simulink library "HANcoder_STM32_Target2009b"  (Simulink 7.5)
settings: Solver=ode45  StartTime=0.0  StopTime=10.0  RelTol=1e-3
libraries: simulink x3
(part 7 of 7)

== system HANcoder_STM32_Target2009b/Olimexino STM32/CAN/CANopenNode/CANopenNode OD Write ==
  In1 : Inport
  S-Function : M-S-Function  FunctionName=sfcn_can_canopennode_od_write  Parameters=tsamp, dataType
  wires:
  In1/1 -> S-Function/1

== system HANcoder_STM32_Target2009b/Olimexino STM32/Memory/EEPROM/Erase EEPROM ==
  Trigger : TriggerPort
  Level-2 M-file S-Function : M-S-Function  FunctionName=sfcn_eeprom_clear

== system HANcoder_STM32_Target2009b/Olimexino STM32/Memory/EEPROM/Read from EEPROM ==
  In1 : Inport
  Level-2 M-file S-Function : M-S-Function  FunctionName=sfcn_eeprom_read  Parameters=tsamp
  Out1 : Outport
  wires:
  In1/1 -> Level-2 M-file S-Function/1
  Level-2 M-file S-Function/1 -> Out1/1

== system HANcoder_STM32_Target2009b/Olimexino STM32/Memory/EEPROM/Save EEPROM ==
  Trigger : TriggerPort
  Level-2 M-file S-Function : M-S-Function  FunctionName=sfcn_eeprom_save

== system HANcoder_STM32_Target2009b/Olimexino STM32/Memory/EEPROM/Write to EEPROM ==
  In1 : Inport
  In2 : Inport  Port=2
  Level-2 M-file S-Function : M-S-Function  FunctionName=sfcn_eeprom_write  Parameters=tsamp
  wires:
  In1/1 -> Level-2 M-file S-Function/1
  In2/1 -> Level-2 M-file S-Function/2

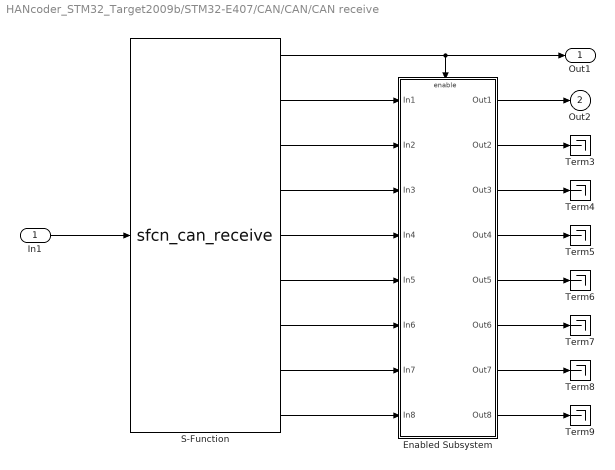
== system HANcoder_STM32_Target2009b/STM32-E407/CAN/CAN/CAN receive ==
  In1 : Inport
  Enabled Subsystem : Subsystem  TreatAsAtomicUnit=on
  S-Function : M-S-Function  FunctionName=sfcn_can_receive  Parameters=tsamp, canBus, outputNumber, dataType, byteOrder
  Term{3..9} (7 alike) : Terminator
  Out1 : Outport
  Out2 : Outport  Port=2
  wires:
  In1/1 -> S-Function/1
  S-Function/1 -> Enabled Subsystem/Enable, Out1/1
  S-Function/2 -> Enabled Subsystem/1(In1)
  S-Function/3 -> Enabled Subsystem/2(In2)
  Enabled Subsystem/1(Out1) -> Out2/1
  Enabled Subsystem/2(Out2) -> Term3/1
  Enabled Subsystem/3(Out3) -> Term4/1
  Enabled Subsystem/4(Out4) -> Term5/1
  Enabled Subsystem/5(Out5) -> Term6/1
  Enabled Subsystem/6(Out6) -> Term7/1
  Enabled Subsystem/7(Out7) -> Term8/1
  Enabled Subsystem/8(Out8) -> Term9/1
  S-Function/6 -> Enabled Subsystem/5(In5)
  S-Function/7 -> Enabled Subsystem/6(In6)
  S-Function/8 -> Enabled Subsystem/7(In7)
  S-Function/5 -> Enabled Subsystem/4(In4)
  S-Function/4 -> Enabled Subsystem/3(In3)
  S-Function/9 -> Enabled Subsystem/8(In8)

== system HANcoder_STM32_Target2009b/STM32-E407/CAN/CAN/CAN receive packed ==
  Enabled Subsystem : Subsystem  TreatAsAtomicUnit=on
  S-Function : M-S-Function  FunctionName=sfcn_can_receive_packed  Parameters=tsamp, canBus, canID
  Out1 : Outport
  Out2 : Outport  Port=2
  wires:
  S-Function/1 -> Enabled Subsystem/Enable, Out1/1
  S-Function/2 -> Enabled Subsystem/1(In1)
  Enabled Subsystem/1(Out1) -> Out2/1

== system HANcoder_STM32_Target2009b/STM32-E407/CAN/CAN/CAN send ==
  In1 : Inport
  In2 : Inport  Port=2
  In3 : Inport  Port=3
  In4 : Inport  Port=4
  In5 : Inport  Port=5
  In6 : Inport  Port=6
  In7 : Inport  Port=7
  In8 : Inport  Port=8
  In9 : Inport  Port=9
  S-Function : M-S-Function  FunctionName=sfcn_can_send  Parameters=tsamp, canBus, frameType, inputNumber, dataType, byteOrder
  wires:
  In9/1 -> S-Function/9
  In8/1 -> S-Function/8
  In7/1 -> S-Function/7
  In6/1 -> S-Function/6
  In5/1 -> S-Function/5
  In4/1 -> S-Function/4
  In3/1 -> S-Function/3
  In2/1 -> S-Function/2
  In1/1 -> S-Function/1

== system HANcoder_STM32_Target2009b/STM32-E407/CAN/CAN/CAN send packed ==
  In1 : Inport
  S-Function : M-S-Function  FunctionName=sfcn_can_send_packed  Parameters=tsamp, canBus
  wires:
  In1/1 -> S-Function/1

== system HANcoder_STM32_Target2009b/STM32-E407/CAN/CANopenNode/CANopenNode Init ==
  S-Function : M-S-Function  FunctionName=sfcn_can_canopennode_init  Parameters=channel

== system HANcoder_STM32_Target2009b/STM32-E407/CAN/CANopenNode/CANopenNode OD Read ==
  S-Function : M-S-Function  FunctionName=sfcn_can_canopennode_od_read  Parameters=tsamp, dataType
  Out1 : Outport
  wires:
  S-Function/1 -> Out1/1

== system HANcoder_STM32_Target2009b/STM32-E407/CAN/CANopenNode/CANopenNode OD Write ==
  In1 : Inport
  S-Function : M-S-Function  FunctionName=sfcn_can_canopennode_od_write  Parameters=tsamp, dataType
  wires:
  In1/1 -> S-Function/1

== system HANcoder_STM32_Target2009b/STM32-E407/Memory/EEPROM/Erase EEPROM ==
  Trigger : TriggerPort
  Level-2 M-file S-Function : M-S-Function  FunctionName=sfcn_eeprom_clear

== system HANcoder_STM32_Target2009b/STM32-E407/Memory/EEPROM/Read from EEPROM ==
  In1 : Inport
  Level-2 M-file S-Function : M-S-Function  FunctionName=sfcn_eeprom_read  Parameters=tsamp
  Out1 : Outport
  wires:
  Level-2 M-file S-Function/1 -> Out1/1
  In1/1 -> Level-2 M-file S-Function/1

== system HANcoder_STM32_Target2009b/STM32-E407/Memory/EEPROM/Save EEPROM ==
  Trigger : TriggerPort
  Level-2 M-file S-Function : M-S-Function  FunctionName=sfcn_eeprom_save

== system HANcoder_STM32_Target2009b/STM32-E407/Memory/EEPROM/Write to EEPROM ==
  In1 : Inport
  In2 : Inport  Port=2
  Level-2 M-file S-Function : M-S-Function  FunctionName=sfcn_eeprom_write  Parameters=tsamp
  wires:
  In2/1 -> Level-2 M-file S-Function/2
  In1/1 -> Level-2 M-file S-Function/1

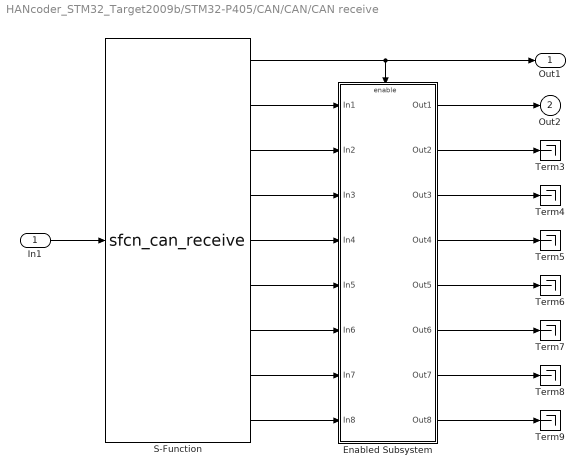
== system HANcoder_STM32_Target2009b/STM32-P405/CAN/CAN/CAN receive ==
  In1 : Inport
  Enabled Subsystem : Subsystem  TreatAsAtomicUnit=on
  S-Function : M-S-Function  FunctionName=sfcn_can_receive  Parameters=tsamp, canBus, outputNumber, dataType, byteOrder
  Term{3..9} (7 alike) : Terminator
  Out1 : Outport
  Out2 : Outport  Port=2
  wires:
  In1/1 -> S-Function/1
  S-Function/1 -> Out1/1, Enabled Subsystem/Enable
  S-Function/2 -> Enabled Subsystem/1(In1)
  S-Function/3 -> Enabled Subsystem/2(In2)
  Enabled Subsystem/1(Out1) -> Out2/1
  Enabled Subsystem/2(Out2) -> Term3/1
  Enabled Subsystem/3(Out3) -> Term4/1
  Enabled Subsystem/4(Out4) -> Term5/1
  Enabled Subsystem/5(Out5) -> Term6/1
  Enabled Subsystem/6(Out6) -> Term7/1
  Enabled Subsystem/7(Out7) -> Term8/1
  Enabled Subsystem/8(Out8) -> Term9/1
  S-Function/6 -> Enabled Subsystem/5(In5)
  S-Function/7 -> Enabled Subsystem/6(In6)
  S-Function/8 -> Enabled Subsystem/7(In7)
  S-Function/5 -> Enabled Subsystem/4(In4)
  S-Function/4 -> Enabled Subsystem/3(In3)
  S-Function/9 -> Enabled Subsystem/8(In8)

== system HANcoder_STM32_Target2009b/STM32-P405/CAN/CAN/CAN receive packed ==
  Enabled Subsystem : Subsystem  TreatAsAtomicUnit=on
  S-Function : M-S-Function  FunctionName=sfcn_can_receive_packed  Parameters=tsamp, canBus, canID
  Out1 : Outport
  Out2 : Outport  Port=2
  wires:
  S-Function/1 -> Enabled Subsystem/Enable, Out1/1
  S-Function/2 -> Enabled Subsystem/1(In1)
  Enabled Subsystem/1(Out1) -> Out2/1

== system HANcoder_STM32_Target2009b/STM32-P405/CAN/CAN/CAN send ==
  In1 : Inport
  In2 : Inport  Port=2
  In3 : Inport  Port=3
  In4 : Inport  Port=4
  In5 : Inport  Port=5
  In6 : Inport  Port=6
  In7 : Inport  Port=7
  In8 : Inport  Port=8
  In9 : Inport  Port=9
  S-Function : M-S-Function  FunctionName=sfcn_can_send  Parameters=tsamp, canBus, frameType, inputNumber, dataType, byteOrder
  wires:
  In1/1 -> S-Function/1
  In2/1 -> S-Function/2
  In3/1 -> S-Function/3
  In4/1 -> S-Function/4
  In5/1 -> S-Function/5
  In6/1 -> S-Function/6
  In7/1 -> S-Function/7
  In8/1 -> S-Function/8
  In9/1 -> S-Function/9

== system HANcoder_STM32_Target2009b/STM32-P405/CAN/CAN/CAN send packed ==
  In1 : Inport
  S-Function : M-S-Function  FunctionName=sfcn_can_send_packed  Parameters=tsamp, canBus
  wires:
  In1/1 -> S-Function/1

== system HANcoder_STM32_Target2009b/STM32-P405/CAN/CANopenNode/CANopenNode Init ==
  S-Function : M-S-Function  FunctionName=sfcn_can_canopennode_init  Parameters=channel

== system HANcoder_STM32_Target2009b/STM32-P405/CAN/CANopenNode/CANopenNode OD Read ==
  S-Function : M-S-Function  FunctionName=sfcn_can_canopennode_od_read  Parameters=tsamp, dataType
  Out1 : Outport
  wires:
  S-Function/1 -> Out1/1

== system HANcoder_STM32_Target2009b/STM32-P405/CAN/CANopenNode/CANopenNode OD Write ==
  In1 : Inport
  S-Function : M-S-Function  FunctionName=sfcn_can_canopennode_od_write  Parameters=tsamp, dataType
  wires:
  In1/1 -> S-Function/1

== system HANcoder_STM32_Target2009b/STM32-P405/Memory/EEPROM/Erase EEPROM ==
  Trigger : TriggerPort
  Level-2 M-file S-Function : M-S-Function  FunctionName=sfcn_eeprom_clear

== system HANcoder_STM32_Target2009b/STM32-P405/Memory/EEPROM/Read from EEPROM ==
  In1 : Inport
  Level-2 M-file S-Function : M-S-Function  FunctionName=sfcn_eeprom_read  Parameters=tsamp
  Out1 : Outport
  wires:
  In1/1 -> Level-2 M-file S-Function/1
  Level-2 M-file S-Function/1 -> Out1/1

== system HANcoder_STM32_Target2009b/STM32-P405/Memory/EEPROM/Save EEPROM ==
  Trigger : TriggerPort
  Level-2 M-file S-Function : M-S-Function  FunctionName=sfcn_eeprom_save

== system HANcoder_STM32_Target2009b/STM32-P405/Memory/EEPROM/Write to EEPROM ==
  In1 : Inport
  In2 : Inport  Port=2
  Level-2 M-file S-Function : M-S-Function  FunctionName=sfcn_eeprom_write  Parameters=tsamp
  wires:
  In1/1 -> Level-2 M-file S-Function/1
  In2/1 -> Level-2 M-file S-Function/2

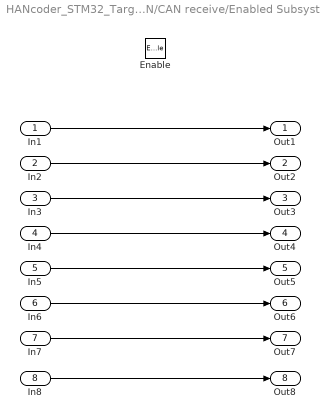
== system HANcoder_STM32_Target2009b/Olimexino STM32/CAN/CAN/CAN receive/Enabled Subsystem ==
  In1 : Inport
  In2 : Inport  Port=2
  In3 : Inport  Port=3
  In4 : Inport  Port=4
  In5 : Inport  Port=5
  In6 : Inport  Port=6
  In7 : Inport  Port=7
  In8 : Inport  Port=8
  Enable : EnablePort
  Out1 : Outport
  Out2 : Outport  Port=2
  Out3 : Outport  Port=3
  Out4 : Outport  Port=4
  Out5 : Outport  Port=5
  Out6 : Outport  Port=6
  Out7 : Outport  Port=7
  Out8 : Outport  Port=8
  wires:
  In1/1 -> Out1/1
  In2/1 -> Out2/1
  In3/1 -> Out3/1
  In4/1 -> Out4/1
  In5/1 -> Out5/1
  In6/1 -> Out6/1
  In7/1 -> Out7/1
  In8/1 -> Out8/1

== system HANcoder_STM32_Target2009b/Olimexino STM32/CAN/CAN/CAN receive packed/Enabled Subsystem ==
  In1 : Inport
  Enable : EnablePort
  Out1 : Outport
  wires:
  In1/1 -> Out1/1

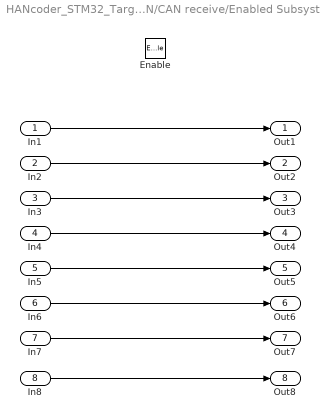
== system HANcoder_STM32_Target2009b/STM32-E407/CAN/CAN/CAN receive/Enabled Subsystem ==
  In1 : Inport
  In2 : Inport  Port=2
  In3 : Inport  Port=3
  In4 : Inport  Port=4
  In5 : Inport  Port=5
  In6 : Inport  Port=6
  In7 : Inport  Port=7
  In8 : Inport  Port=8
  Enable : EnablePort
  Out1 : Outport
  Out2 : Outport  Port=2
  Out3 : Outport  Port=3
  Out4 : Outport  Port=4
  Out5 : Outport  Port=5
  Out6 : Outport  Port=6
  Out7 : Outport  Port=7
  Out8 : Outport  Port=8
  wires:
  In1/1 -> Out1/1
  In2/1 -> Out2/1
  In3/1 -> Out3/1
  In4/1 -> Out4/1
  In5/1 -> Out5/1
  In6/1 -> Out6/1
  In7/1 -> Out7/1
  In8/1 -> Out8/1

== system HANcoder_STM32_Target2009b/STM32-E407/CAN/CAN/CAN receive packed/Enabled Subsystem ==
  In1 : Inport
  Enable : EnablePort
  Out1 : Outport
  wires:
  In1/1 -> Out1/1

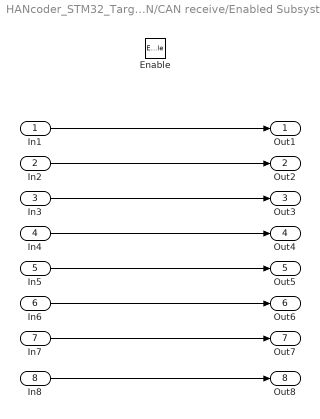
== system HANcoder_STM32_Target2009b/STM32-P405/CAN/CAN/CAN receive/Enabled Subsystem ==
  In1 : Inport
  In2 : Inport  Port=2
  In3 : Inport  Port=3
  In4 : Inport  Port=4
  In5 : Inport  Port=5
  In6 : Inport  Port=6
  In7 : Inport  Port=7
  In8 : Inport  Port=8
  Enable : EnablePort
  Out1 : Outport
  Out2 : Outport  Port=2
  Out3 : Outport  Port=3
  Out4 : Outport  Port=4
  Out5 : Outport  Port=5
  Out6 : Outport  Port=6
  Out7 : Outport  Port=7
  Out8 : Outport  Port=8
  wires:
  In1/1 -> Out1/1
  In2/1 -> Out2/1
  In3/1 -> Out3/1
  In4/1 -> Out4/1
  In5/1 -> Out5/1
  In6/1 -> Out6/1
  In7/1 -> Out7/1
  In8/1 -> Out8/1

== system HANcoder_STM32_Target2009b/STM32-P405/CAN/CAN/CAN receive packed/Enabled Subsystem ==
  In1 : Inport
  Enable : EnablePort
  Out1 : Outport
  wires:
  In1/1 -> Out1/1
